simulink library "Chassis_Alpha_sm"  (R2014a)
settings: Solver=ode45  StartTime=0.0  StopTime=10.0  RelTol=1e-3
undefined symbols (not defined in the file or in its folder): Chassis, X, Y, Z
libraries: sm_lib x6, nesl_utility x5, Chassis_Alpha x2, simulink x2, Chassis_Alpha_sm x1
Description:
  | Copyright 2013-2014 The MathWorks, Inc.
settings Model: Creator=mbrauer  LastModifiedBy=mbrauer

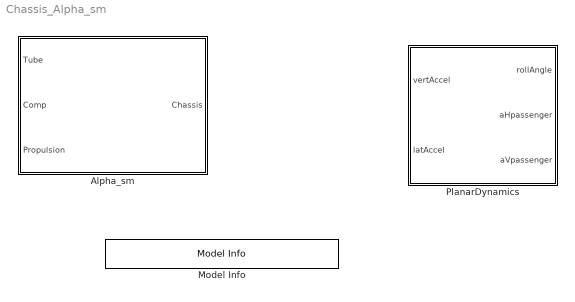
== system Chassis_Alpha_sm ==
  Alpha_sm : Subsystem
  Model Info : simulink/Model-Wide Utilities/Model Info  InitialBlockCM=None  BlockCM=none  Frame=on  DisplayStringWithTags=%<Description>  HorizontalTextAlignment=Center  LeftAlignmentValue=0.5  SourceBlockDiagram=Chassis_Alpha_sm  TagMaxNumber=20
  PlanarDynamics : Subsystem  mask(Upper Link){R=Chassis.TubeRadius, cH=Chassis.Height, cW=Chassis.Width, M=Chassis.Mass, D=5e3 % magic number}
      mask prompts: R "Tube Radius (m)"; cH "Chass height (m):"; cW "Chassis width (m):"; M "Chassis mass (kg)"; D "Damping (N/rad/s)"
      mask help: Upper link of the double pendulum mechanism
      mask init:
      | % Solve trigonmetry to determine chassis location.
      | % Assumes point contact at bottom edges with tube.
      | Alpha  = sqrt(R^2-(cW/2)^2);
      | AirGap = R-Alpha;

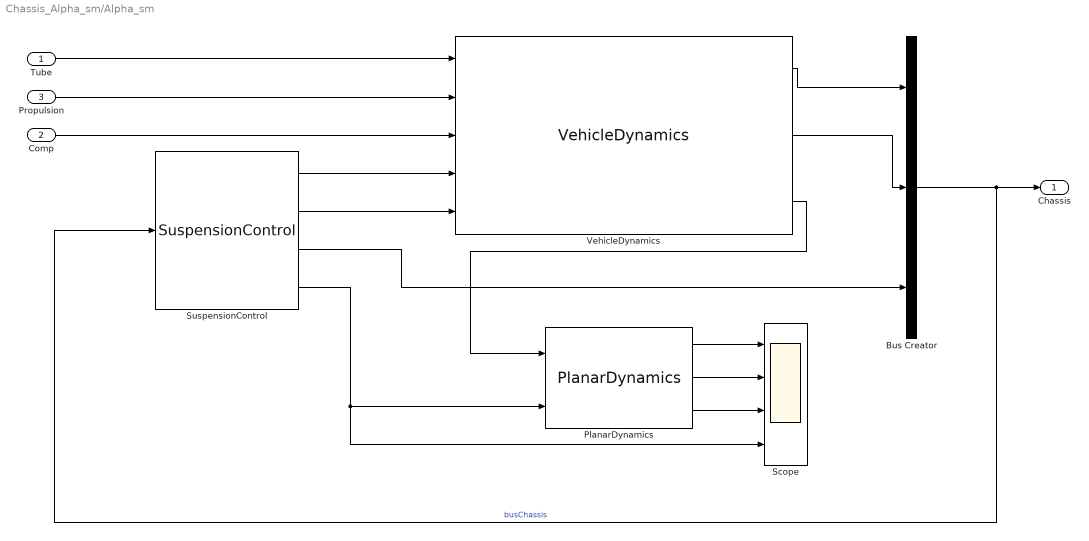
== system Chassis_Alpha_sm/Alpha_sm ==
  "Tube " : Inport
  Comp : Inport  Port=2
  Propulsion : Inport  Port=3
  Bus Creator : BusCreator  Inputs=3  NonVirtualBus=on
  PlanarDynamics : Chassis_Alpha_sm/PlanarDynamics  R=Chassis.TubeRadius  cH=Chassis.Height  cW=Chassis.Width  M=Chassis.Mass  D=5e3 % magic number
  Scope : Scope  NumInputPorts=4
      settings: YMin=-0.1~-12~-9.9~-5  YMax=0.55~2~-8.4~5  Decimation=10
  SuspensionControl : Chassis_Alpha/SuspensionControl
  VehicleDynamics : Chassis_Alpha/VehicleDynamics
  Chassis : Outport
  wires:
  VehicleDynamics/3 -> PlanarDynamics/1
  SuspensionControl/3 -> Bus Creator/3
  SuspensionControl/2 -> VehicleDynamics/5
  SuspensionControl/1 -> VehicleDynamics/4
  Propulsion/1 -> VehicleDynamics/2
  VehicleDynamics/2 -> Bus Creator/2
  VehicleDynamics/1 -> Bus Creator/1
  "Tube "/1 -> VehicleDynamics/1
  Comp/1 -> VehicleDynamics/3
  Bus Creator/1 -> Chassis/1, SuspensionControl/1  "busChassis"
  SuspensionControl/4 -> PlanarDynamics/2, Scope/4
  PlanarDynamics/1 -> Scope/1
  PlanarDynamics/2 -> Scope/2
  PlanarDynamics/3 -> Scope/3

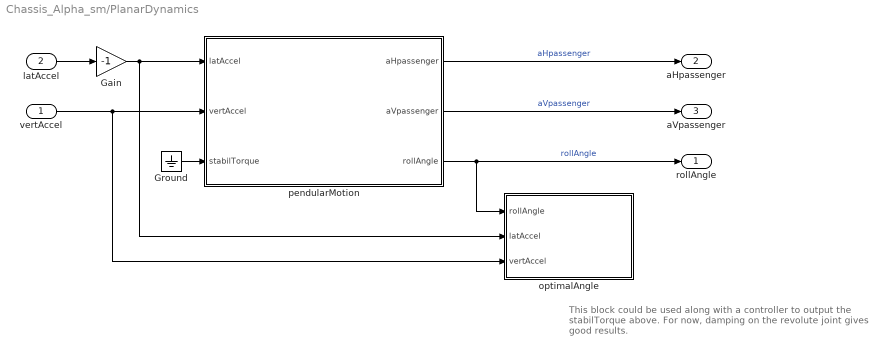
== system Chassis_Alpha_sm/PlanarDynamics ==
  note: This block could be used along with a
      | controller to output the stabilTorque above.
      |
      | For now, damping on the revolute joint gives good results.
  vertAccel : Inport
  latAccel : Inport  Port=2
  Gain : Gain  Gain=-1
  Ground : Ground
  optimalAngle : Subsystem
  pendularMotion : Subsystem
  rollAngle : Outport
  aHpassenger : Outport  Port=2
  aVpassenger : Outport  Port=3
  wires:
  Ground/1 -> pendularMotion/3(stabilTorque)
  vertAccel/1 -> pendularMotion/2(vertAccel), optimalAngle/3(vertAccel)
  Gain/1 -> pendularMotion/1(latAccel), optimalAngle/2(latAccel)
  pendularMotion/2(aVpassenger) -> aVpassenger/1  "aVpassenger"
  pendularMotion/1(aHpassenger) -> aHpassenger/1  "aHpassenger"
  pendularMotion/3(rollAngle) -> rollAngle/1, optimalAngle/1(rollAngle)  "rollAngle"
  latAccel/1 -> Gain/1

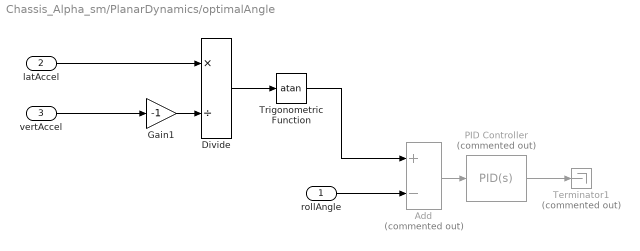
== system Chassis_Alpha_sm/PlanarDynamics/optimalAngle ==
  rollAngle : Inport
  latAccel : Inport  Port=2
  vertAccel : Inport  Port=3
  Add : Sum  Commented=on  Inputs=+-
  Divide : Product  Inputs=*/
  Gain1 : Gain  Gain=-1
  PID Controller : simulink/Continuous/PID Controller  Commented=on  Controller=PID  TimeDomain=Continuous-time  SampleTime=1  IntegratorMethod=Forward Euler  FilterMethod=Forward Euler  Form=Parallel  P=0 % 1.50e5  I=0 % 2.8e5  D=0 % 1.8e4  N=65  InitialConditionSource=internal  InitialConditionForIntegrator=0  InitialConditionForFilter=0  ExternalReset=none  LimitOutput=off  UpperSaturationLimit=inf  LowerSaturationLimit=-inf  LinearizeAsGain=on  AntiWindupMode=none  Kb=1  TrackingMode=off  Kt=1  PParamMin=[]  PParamMax=[]  IParamMin=[]  IParamMax=[]  DParamMin=[]  DParamMax=[]  NParamMin=[]  NParamMax=[]  KbParamMin=[]  KbParamMax=[]  KtParamMin=[]  KtParamMax=[]  POutMin=[]  POutMax=[]  IOutMin=[]  IOutMax=[]  DOutMin=[]  DOutMax=[]  NOutMin=[]  NOutMax=[]  KbOutMin=[]  KbOutMax=[]  KtOutMin=[]  KtOutMax=[]  IntegratorOutMin=[]  IntegratorOutMax=[]  FilterOutMin=[]  FilterOutMax=[]  SumOutMin=[]  SumOutMax=[]  SumI1OutMin=[]  SumI1OutMax=[]  SumI2OutMin=[]  SumI2OutMax=[]  SumI3OutMin=[]  SumI3OutMax=[]  SumDOutMin=[]  SumDOutMax=[]  SaturationOutMin=[]  SaturationOutMax=[]  IntegratorContinuousStateAttributes=''  IntegratorStateMustResolveToSignalObject=off  IntegratorRTWStateStorageClass=Auto  FilterContinuousStateAttributes=''  FilterStateMustResolveToSignalObject=off  FilterRTWStateStorageClass=Auto
  Terminator1 : Terminator  Commented=on
  Trigonometric Function : Trigonometry  Operator=atan
  wires:
  rollAngle/1 -> Add/2
  PID Controller/1 -> Terminator1/1
  Trigonometric Function/1 -> Add/1
  Add/1 -> PID Controller/1
  latAccel/1 -> Divide/1
  vertAccel/1 -> Gain1/1
  Gain1/1 -> Divide/2
  Divide/1 -> Trigonometric Function/1

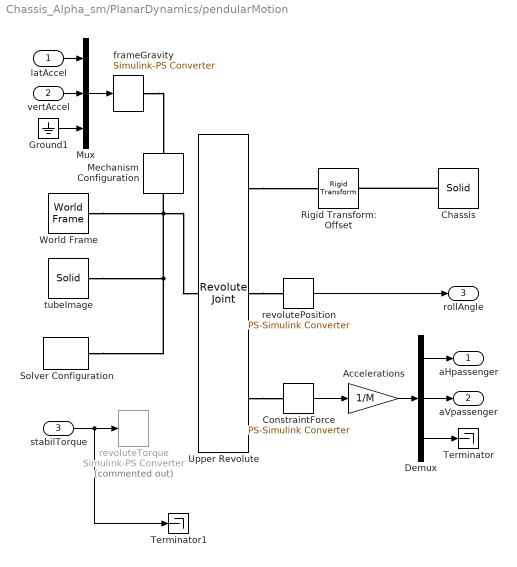
== system Chassis_Alpha_sm/PlanarDynamics/pendularMotion ==
  latAccel : Inport
  vertAccel : Inport  Port=2
  stabilTorque : Inport  Port=3
  Accelerations : Gain  Gain=1/M
  Chassis : sm_lib/Body Elements/Solid  InertiaType=PointMass  Mass=M  MassUnits=kg  CenterOfMass=[0 0 0]  CenterOfMassUnits=m  MomentsOfInertia=[1 1 1]  MomentsOfInertiaUnits=kg*m^2  ProductsOfInertia=[0 0 0]  ProductsOfInertiaUnits=kg*m^2  DensityBased=on  Density=1  DensityUnits=kg/m^3  GraphicType=FromGeometry  MarkerShape=Sphere  MarkerSize=1  MarkerSizeUnits=m  GraphicVisPropType=SimpleVisualProperties  GraphicDiffuseColor=[0.2 0.4 1.0]  GraphicSpecularColor=[0.2 0.2 0.2]  GraphicAmbientColor=[0.5 0.5 0.5]  GraphicEmissiveColor=[0.1 0.1 0.1]  GraphicShininess=24.0  GraphicOpacity=1  GeometryShape=Brick  RectangleSize=[1 1]  RectangleSizeUnits=m  BrickDimensions=[cW cH 1]  BrickDimensionUnits=m  CylinderRadius=1  CylinderRadiusUnits=cm  CylinderLength=1  CylinderLengthUnits=cm  SphereRadius=1  SphereRadiusUnits=m  EllipsoidRadii=[1 1 1]  EllipsoidRadiiUnits=m  ExtrusionCrossSection=[1 1; -1 1; -1 -1; 1 -1]  ExtrusionCrossSectionUnits=m  ExtrusionLength=1  ExtrusionLengthUnits=m  PolygonNumSides=1  PolygonOuterRadius=1  PolygonOuterRadiusUnits=m  ExtGeomFileType=STL  ExtGeomFileUnits=m  RevolutionCrossSection=[1 1; 1 -1; 2 -1; 2 1]  RevolutionCrossSectionUnits=m  RevolutionExtent=Full  RevolutionAngle=180  RevolutionAngleUnits=deg  BlockFunction=simmechanics.library.body_elements.solid
      settings: AttributesFormatString=|
      | Mass = %<Mass>
      | %<BrickDimensions>
  ConstraintForce : nesl_utility/PS-Simulink Converter  PhysicalDomain=network_engine_domain  SubClassName=ps_output  LeftPortType=input  RightPortType=output  PseudoPeriodic=off  Frequencies=[]  Unit=N  AffineConversion=off
  Demux : Demux  Outputs=3
  Ground1 : Ground
  Mechanism Configuration : sm_lib/Utilities/Mechanism Configuration  UniformGravity=TimeVarying  GravityVector=[0 0 -9.80665]  GravityUnits=m/s^2  LinearizationDelta=0.001  BlockFunction=simmechanics.library.utilities.mechanism_configuration
  Mux : Mux  Inputs=3
  Rigid Transform: Offset : sm_lib/Frames and Transforms/Rigid Transform  TranslationMethod=Cartesian  TranslationLengthUnit=m  TranslationStandardAxis=+Z  TranslationStandardOffset=0  TranslationCartesianOffset=[0 cH/2-sqrt(R^2-(cW/2)^2) 0]  TranslationROffset=0  TranslationROffsetUnits=m  TranslationZOffset=0  TranslationZOffsetUnits=m  TranslationThetaOffset=0  TranslationThetaOffsetUnits=deg  RotationMethod=None  RotationAngleUnits=deg  RotationStandardAxis=+Z  RotationAngle=0  RotationArbitraryAxis=[0 0 1]  FollAlignAxisA=+X  BaseAlignAxisA=+Y  FollAlignAxisB=+Y  BaseAlignAxisB=+Z  BlockFunction=simmechanics.library.frames_transforms.rigid_transform
      settings: AttributesFormatString=|
      | Trans Method: %<TranslationMethod>
      | %<TranslationCartesianOffset>
  Solver Configuration : nesl_utility/Solver Configuration  PhysicalDomain=network_engine_domain  SubClassName=solver  LeftPortType=input  RightPortType=generic  Accelerate=off  Tones=[]  Harmonics=[]  SimulateNoise=off  Profile=off  UseLocalSampling=off  EnableSwitchedLinearOptims=on  FrequencyDomain=off  UseCCode=off  RelTol=0.001  AbsTol=1e-06  MinStep=1e-09  ToWorkspace=off  DoDC=off  ResidualTolerance=1e-9  UseLocalSolver=off  LocalSolverChoice=NE_BACKWARD_EULER_ADVANCER  LocalSolverSampleTime=.001  DoFixedCost=off  MaxNonlinIter=3  MaxModeIter=2  LinearAlgebra=Sparse  DelaysMemoryBudget=1024  AutomaticFiltering=on  FilteringTimeConstant=0.001
  Terminator : Terminator
  Terminator1 : Terminator
  Upper Revolute : sm_lib/Joints/Revolute Joint  SenseConstraintForce=on  SenseConstraintForceX=off  SenseConstraintForceY=off  SenseConstraintForceZ=off  SenseConstraintTorque=off  SenseConstraintTorqueX=off  SenseConstraintTorqueY=off  SenseConstraintTorqueZ=off  SenseTotalForce=off  SenseTotalForceX=off  SenseTotalForceY=off  SenseTotalForceZ=off  SenseTotalTorque=off  SenseTotalTorqueX=off  SenseTotalTorqueY=off  SenseTotalTorqueZ=off  CompositeWrenchDir=FollowerOnBase  CompositeWrenchFrame=FollowerFrame  EquilibriumPosition=0  EquilibriumPositionUnits=rad  SpringStiffness=0  SpringStiffnessUnits=N*m/rad  DampingCoefficient=D  DampingCoefficientUnits=N*m/(rad/s)  TorqueActuationMode=NoTorque  MotionActuationMode=ComputedMotion  SensePosition=on  SenseVelocity=off  SenseAcceleration=off  SenseTorqueForce=off  PositionTargetValue=0  PositionTargetValueUnits=deg  PositionTargetSpecify=on  PositionTargetPriority=High  VelocityTargetValue=0  VelocityTargetValueUnits=rad/s  VelocityTargetSpecify=off  VelocityTargetPriority=Low  BlockFunction=simmechanics.library.joints.revolute_joint
  World Frame : sm_lib/Frames and Transforms/World Frame  BlockFunction=simmechanics.library.frames_transforms.world_frame
  frameGravity : nesl_utility/Simulink-PS Converter  PhysicalDomain=network_engine_domain  SubClassName=ps_input  LeftPortType=input  RightPortType=output  PseudoPeriodic=off  Frequencies=[]  NoiseDistribution=none  NoiseParameters=[]  Unit=m/s^2  AffineConversion=off  InputFiltering=off  SimscapeFilterOrder=1  InputFilterTimeConstant=0.001  UdotUserProvided=1
  revolutePosition : nesl_utility/PS-Simulink Converter  PhysicalDomain=network_engine_domain  SubClassName=ps_output  LeftPortType=input  RightPortType=output  PseudoPeriodic=off  Frequencies=[]  Unit=rad  AffineConversion=off
  revoluteTorque : nesl_utility/Simulink-PS Converter  Commented=on  PhysicalDomain=network_engine_domain  SubClassName=ps_input  LeftPortType=input  RightPortType=output  PseudoPeriodic=off  Frequencies=[]  NoiseDistribution=none  NoiseParameters=[]  Unit=N*m  AffineConversion=off  InputFiltering=off  SimscapeFilterOrder=1  InputFilterTimeConstant=0.001  UdotUserProvided=1
  tubeImage : sm_lib/Body Elements/Solid  InertiaType=PointMass  Mass=1  MassUnits=kg  CenterOfMass=[0 0 0]  CenterOfMassUnits=m  MomentsOfInertia=[1 1 1]  MomentsOfInertiaUnits=kg*m^2  ProductsOfInertia=[0 0 0]  ProductsOfInertiaUnits=kg*m^2  DensityBased=on  Density=1  DensityUnits=kg/m^3  GraphicType=FromGeometry  MarkerShape=Sphere  MarkerSize=1  MarkerSizeUnits=m  GraphicVisPropType=SimpleVisualProperties  GraphicDiffuseColor=[0.6 0.6 0.6]  GraphicSpecularColor=[0.2 0.2 0.2]  GraphicAmbientColor=[0.5 0.5 0.5]  GraphicEmissiveColor=[0.1 0.1 0.1]  GraphicShininess=24.0  GraphicOpacity=1  GeometryShape=Cylinder  RectangleSize=[1 1]  RectangleSizeUnits=m  BrickDimensions=[cW cH 1]  BrickDimensionUnits=m  CylinderRadius=R  CylinderRadiusUnits=m  CylinderLength=1  CylinderLengthUnits=cm  SphereRadius=1  SphereRadiusUnits=m  EllipsoidRadii=[1 1 1]  EllipsoidRadiiUnits=m  ExtrusionCrossSection=[1 1; -1 1; -1 -1; 1 -1]  ExtrusionCrossSectionUnits=m  ExtrusionLength=1  ExtrusionLengthUnits=m  PolygonNumSides=1  PolygonOuterRadius=1  PolygonOuterRadiusUnits=m  ExtGeomFileType=STL  ExtGeomFileUnits=m  RevolutionCrossSection=[1 1; 1 -1; 2 -1; 2 1]  RevolutionCrossSectionUnits=m  RevolutionExtent=Full  RevolutionAngle=180  RevolutionAngleUnits=deg  BlockFunction=simmechanics.library.body_elements.solid
      settings: AttributesFormatString=CylinderRadius = %<CylinderRadius>
  aHpassenger : Outport
  aVpassenger : Outport  Port=2
  rollAngle : Outport  Port=3
  wires:
  stabilTorque/1 -> revoluteTorque/1, Terminator1/1
  Mux/1 -> frameGravity/1
  Ground1/1 -> Mux/3
  vertAccel/1 -> Mux/2
  latAccel/1 -> Mux/1
  Accelerations/1 -> Demux/1
  Demux/3 -> Terminator/1
  Demux/1 -> aHpassenger/1
  Demux/2 -> aVpassenger/1
  ConstraintForce/1 -> Accelerations/1
  revolutePosition/1 -> rollAngle/1
  connections:
  frameGravity/RConn1 -- Mechanism Configuration/LConn1
  Chassis/RConn1 -- Rigid Transform: Offset/RConn1
  Upper Revolute/RConn3 -- ConstraintForce/LConn1
  Upper Revolute/RConn1 -- Rigid Transform: Offset/LConn1
  Upper Revolute/RConn2 -- revolutePosition/LConn1
  tubeImage/RConn1 -- Solver Configuration/RConn1 -- Upper Revolute/LConn1 -- Mechanism Configuration/RConn1 -- World Frame/RConn1
